simulink model "DC_Motor_Model"  (R2023b)
settings: Solver=VariableStepAuto  StartTime=0.0  StopTime=20  RelTol=1e-3
InitFcn:
  | Jm=0.000052;
  | Bm=0.01;
  | Kb=0.235;
  | Kt=0.235;
  | Ra=2;
  | La=0.23

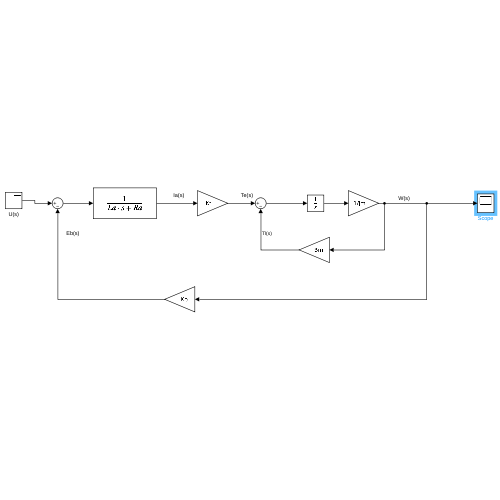
[thumbnail: Simulink's stored preview of the top-level diagram]
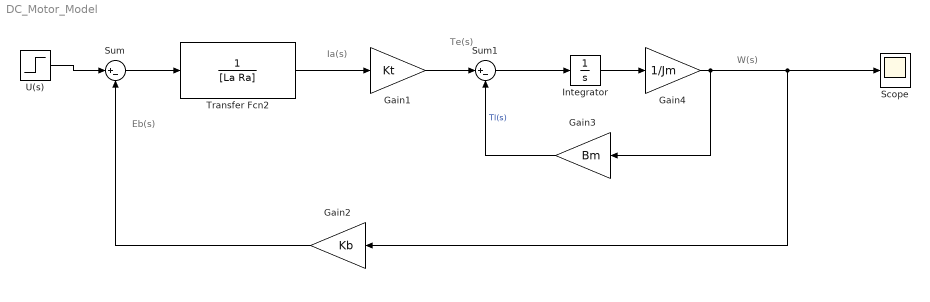
== system DC_Motor_Model ==
  note: Eb(s)
  note: W(s)
  note: Te(s)
  note: Ia(s)
  Gain1 : Gain  Gain=Kt
  Gain2 : Gain  Gain=Kb
  Gain3 : Gain  Gain=Bm
  Gain4 : Gain  Gain=1/Jm
  Integrator : Integrator
  Scope : Scope
  Sum : Sum  Inputs=|+-
  Sum1 : Sum  Inputs=|+-
  Transfer Fcn2 : TransferFcn  Denominator=[La Ra]
  U(s) : Step  Time=2  After=10  SampleTime=0
  wires:
  Sum/1 -> Transfer Fcn2/1
  Transfer Fcn2/1 -> Gain1/1
  Gain2/1 -> Sum/2
  Gain1/1 -> Sum1/1
  Sum1/1 -> Integrator/1
  Integrator/1 -> Gain4/1
  Gain4/1 -> Gain3/1, Gain2/1, Scope/1
  Gain3/1 -> Sum1/2  "Tl(s)"
  U(s)/1 -> Sum/1
